simulink subsystem "DMPC"  (R2023a)
settings: Solver=VariableStepAuto  StartTime=0.0  StopTime=10.0  RelTol=1e-3
settings Model: Creator=giaco  LastModifiedBy=giaco

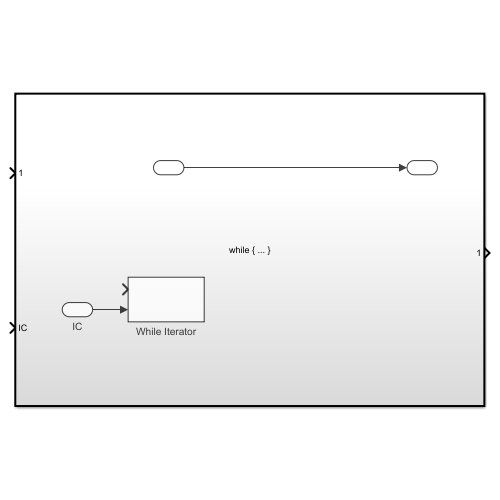
[thumbnail: Simulink's stored preview of the top-level diagram]
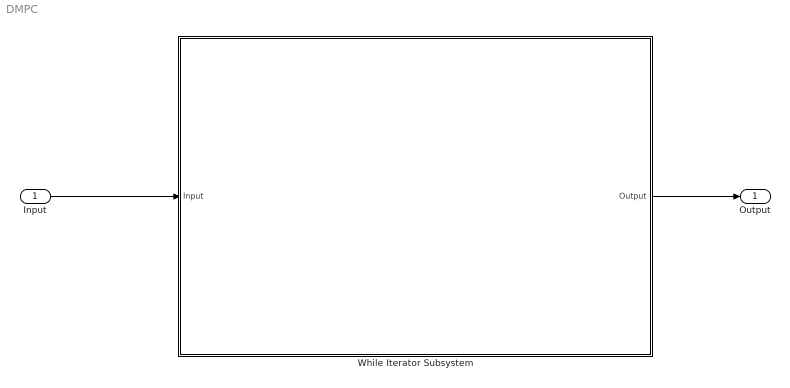
== system DMPC ==
  Input : Inport
  While Iterator Subsystem : Subsystem  TreatAsAtomicUnit=on
  Output : Outport
  wires:
  Input/1 -> While Iterator Subsystem/1(Input)
  While Iterator Subsystem/1(Output) -> Output/1

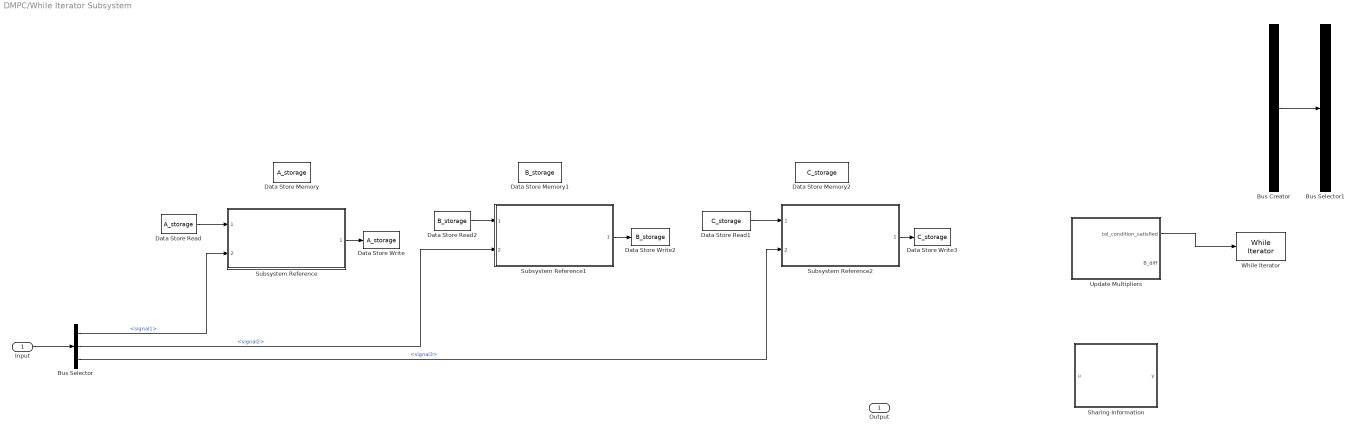
== system DMPC/While Iterator Subsystem ==
  Input : Inport
  Bus Creator : BusCreator  Inputs=9
  Bus Selector : BusSelector  OutputSignals=signal1,signal2,signal3
  Bus Selector1 : BusSelector  OutputSignals=signal1,signal2,signal1,signal2,signal3,signal4,signal5,signal6,signal7,signal8,signal9
  Data Store Memory : DataStoreMemory  DataStoreName=A_storage  WriteAfterWriteMsg=warning  ShowAdditionalParam=off
  Data Store Memory1 : DataStoreMemory  DataStoreName=B_storage  WriteAfterWriteMsg=warning  ShowAdditionalParam=off
  Data Store Memory2 : DataStoreMemory  DataStoreName=C_storage  WriteAfterWriteMsg=warning  ShowAdditionalParam=off
  Data Store Read : DataStoreRead  DataStoreName=A_storage  IndexOptions=Index vector (dialog)  Indices=1  OutputSizes=1
  Data Store Read1 : DataStoreRead  DataStoreName=C_storage  IndexOptions=Index vector (dialog)  Indices=1  OutputSizes=1
  Data Store Read2 : DataStoreRead  DataStoreName=B_storage  IndexOptions=Index vector (dialog)  Indices=1  OutputSizes=1
  Data Store Write : DataStoreWrite  DataStoreName=A_storage  IndexOptions=Index vector (dialog)  Indices=1  OutputSizes=1
  Data Store Write2 : DataStoreWrite  DataStoreName=B_storage  IndexOptions=Index vector (dialog)  Indices=1  OutputSizes=1
  Data Store Write3 : DataStoreWrite  DataStoreName=C_storage  IndexOptions=Index vector (dialog)  Indices=1  OutputSizes=1
  Sharing Information : MATLAB Function  TreatAsAtomicUnit=on
  Subsystem Reference : Subsystem  ReferencedSubsystem=FirstHouse
  Subsystem Reference1 : Subsystem  ReferencedSubsystem=MiddleHouse
  Subsystem Reference2 : Subsystem  ReferencedSubsystem=BypassHouse
  Update Multipliers : MATLAB Function  TreatAsAtomicUnit=on
  While Iterator : WhileIterator  MaxIters=1000  WhileBlockType=do-while
  Output : Outport
  wires:
  Update Multipliers/1(tol_condition_satisfied) -> While Iterator/1
  Bus Creator/1 -> Bus Selector1/1
  Subsystem Reference/1 -> Data Store Write/1
  Data Store Read/1 -> Subsystem Reference/1
  Input/1 -> Bus Selector/1
  Bus Selector/3 -> Subsystem Reference2/2  "<signal3>"
  Bus Selector/2 -> Subsystem Reference1/2  "<signal2>"
  Subsystem Reference2/1 -> Data Store Write3/1
  Bus Selector/1 -> Subsystem Reference/2  "<signal1>"
  Subsystem Reference1/1 -> Data Store Write2/1
  Data Store Read2/1 -> Subsystem Reference1/1
  Data Store Read1/1 -> Subsystem Reference2/1

== matlab function DMPC/While Iterator Subsystem/Sharing Information ==
  data: u input; y output
function y = fcn(u)

y = u;

== matlab function DMPC/While Iterator Subsystem/Update Multipliers ==
  data: tol_condition_satisfied output boolean; C_storage data_store_memory; B_storage data_store_memory; A_storage data_store_memory; B_diff output
function [tol_condition_satisfied, B_diff] = fcn

global A_storage
global B_storage
global C_storage

persistent difference
if isempty(difference)
    difference = struct();
end

TOL = 1;

% Copy update
B_storage.B.m_O_pred_pred = A_storage.A.mv.m_out_I_I;
% Difference
difference.B.m_out_pred_I = (B_storage.mv.m_out_pred_I - B_storage.B.m_O_pred_pred);
% Multiplier update
B_storage.B.delta_m_O_pred = B_storage.B.delta_m_O_pred + B_storage.B.alfa_m_O_pred * difference.B.m_out_pred_I;


if sum(difference.B.m_out_pred_I) <= TOL
    tol_condition_satisfied = true;
else
    tol_condition_satisfied = false;
end
